simulink model "ps7"  (R2020b)
settings: Solver=VariableStepAuto  StartTime=0.0  StopTime=10.0  RelTol=1e-3
settings Model: Creator=prana  LastModifiedBy=prana

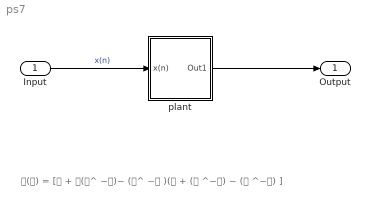
== system ps7 ==
  note: 𝐇(𝐳) = [𝟏 + 𝟐(𝐳^ −𝟏)− (𝐳^ −𝟐 )(𝟏 + (𝐳 ^−𝟏) − (𝐳 ^−𝟐) ]
  Input : Inport
  plant : Subsystem
  Output : Outport
  wires:
  Input/1 -> plant/1(x(n))  "x(n)"
  plant/1(Out1) -> Output/1

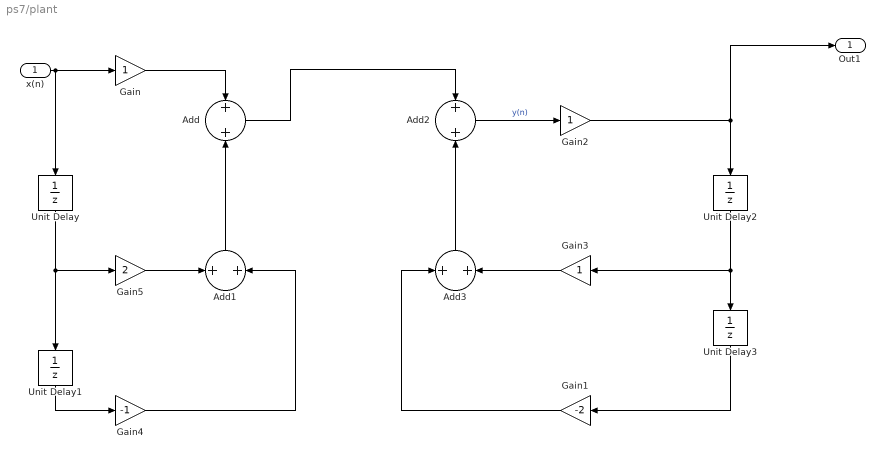
== system ps7/plant ==
  x(n) : Inport
  Add{,1..3} (4 alike) : Sum
  Gain : Gain
  Gain1 : Gain  Gain=-2
  Gain2 : Gain
  Gain3 : Gain
  Gain4 : Gain  Gain=-1
  Gain5 : Gain  Gain=2
  Unit Delay{,1..3} (4 alike) : UnitDelay  SampleTime=-1  HasFrameUpgradeWarning=on
  Out1 : Outport
  wires:
  Add3/1 -> Add2/2
  Unit Delay2/1 -> Gain3/1, Unit Delay3/1
  Add/1 -> Add2/1
  Unit Delay3/1 -> Gain1/1
  Add2/1 -> Gain2/1  "y(n)"
  Unit Delay/1 -> Gain5/1, Unit Delay1/1
  Unit Delay1/1 -> Gain4/1
  Add1/1 -> Add/2
  Gain5/1 -> Add1/1
  Gain3/1 -> Add3/2
  Gain1/1 -> Add3/1
  Gain2/1 -> Out1/1, Unit Delay2/1
  Gain4/1 -> Add1/2
  Gain/1 -> Add/1
  x(n)/1 -> Unit Delay/1, Gain/1
